simulink model "Assignment_3"  (R2020b)
settings: Solver=VariableStepAuto  StartTime=0.0  StopTime=25  RelTol=1e-3
InitFcn:
  | g = 32.18;
  | v0 = 88;
  | Rr = 15/12;
  | Kf = 1;
  | m = 50;
  | PBmax = 1500;
  | TB = 0.01;
  | I = 5;
  | 
  | 
  | ctrl = 1;
settings Model: Creator=Shantam Garg  LastModifiedBy=Shantam Garg

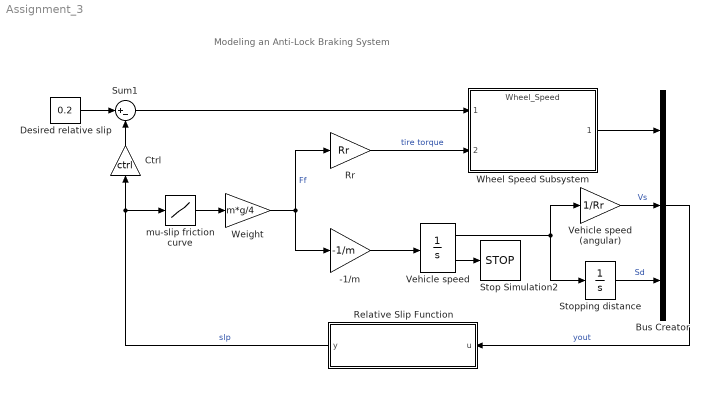
== system Assignment_3 ==
  note: Modeling an Anti-Lock Braking System
  -1/m : Gain  Gain=-1/m  SaturateOnIntegerOverflow=on  OutDataTypeStr=Inherit: Same as input  ParamDataTypeStr=Inherit: Same as input
  Bus Creator : BusCreator  Inputs=3
  Ctrl : Gain  Gain=ctrl  SaturateOnIntegerOverflow=on  OutDataTypeStr=Inherit: Same as input  ParamDataTypeStr=Inherit: Same as input
  Desired relative slip : Constant  Value=0.2
  Relative Slip Function : MATLAB Function  TreatAsAtomicUnit=on
  Rr : Gain  Gain=Rr  SaturateOnIntegerOverflow=on  OutDataTypeStr=Inherit: Same as input  ParamDataTypeStr=Inherit: Same as input
  Stop Simulation2 : Stop
  Stopping distance : Integrator  UpperSaturationLimit=1000  LowerSaturationLimit=0
  Sum1 : Sum  Inputs=|+-  InputSameDT=on  SaturateOnIntegerOverflow=on  OutDataTypeStr=Inherit: Same as first input
  Vehicle speed : Integrator  InitialCondition=v0  LimitOutput=on  UpperSaturationLimit=1000  LowerSaturationLimit=0  ShowSaturationPort=on
  Vehicle speed (angular) : Gain  Gain=1/Rr  SaturateOnIntegerOverflow=on  OutDataTypeStr=Inherit: Same as input  ParamDataTypeStr=Inherit: Same as input
  Weight : Gain  Gain=m*g/4  SaturateOnIntegerOverflow=on  OutDataTypeStr=Inherit: Same as input  ParamDataTypeStr=Inherit: Same as input
  Wheel Speed Subsystem : ModelReference  ModelNameDialog=Wheel_Speed  SimulationMode=Normal  ModelReferenceVersion=1.6
  mu-slip friction curve : Lookup_n-D  NumberOfTableDimensions=1  BreakpointsForDimension1=[0:.05:1.0]  Table=[0 .4 .8 .97 1.0 .98 .96 .94 .92 .9 .88 .855 .83 .81 .79 .77 .75 .73 .72 .71 .7]  SaturateOnIntegerOverflow=on  InputSameDT=on
  wires:
  Vehicle speed/1 -> Stopping distance/1, Vehicle speed (angular)/1
  -1/m/1 -> Vehicle speed/1
  mu-slip friction curve/1 -> Weight/1
  Weight/1 -> -1/m/1, Rr/1  "Ff"
  Desired relative slip/1 -> Sum1/1
  Stopping distance/1 -> Bus Creator/3  "Sd"
  Bus Creator/1 -> Relative Slip Function/1(u)  "yout"
  Vehicle speed/2 -> Stop Simulation2/1
  Ctrl/1 -> Sum1/2
  Vehicle speed (angular)/1 -> Bus Creator/2  "Vs"
  Sum1/1 -> Wheel Speed Subsystem/1
  Rr/1 -> Wheel Speed Subsystem/2  "tire torque"
  Wheel Speed Subsystem/1 -> Bus Creator/1
  Relative Slip Function/1(y) -> mu-slip friction curve/1, Ctrl/1  "slp"

== matlab function Assignment_3/Relative Slip Function ==
  data: u input; y output
function y = Relative_Slip(u)
u = 1.0 - u(1)/(u(2) + (u(2)==0)*eps);
y = u;
